simulink model "test_init"  (Simulink 10.0)
settings: Solver=FixedStepDiscrete  StartTime=0.0  StopTime=100.0  FixedStep=1  RelTol=1e-3  EnableMultiTasking=on
settings Model: Creator=kbrotman  LastModifiedBy=celit
settings DataIOCC: LimitDataPoints=on  SignalLoggingSaveFormat=ModelDataLogs  SignalLoggingName=sigsOut
settings OptimizationCC: LifeSpan=auto
settings DebuggingCC: SaveWithParameterizedLinksMsg=none  UnderspecifiedInitializationDetection=Simplified  SignalResolutionControl=TryResolveAllWithWarning  MultiTaskDSMMsg=warning  MultiTaskCondExecSysMsg=none  SFUnexpectedBacktrackingDiag=error  SFNoUnconditionalDefaultTransitionDiag=error  SFExecutionAtInitializationDiag=warning  ArithmeticOperatorsInVariantConditions=error
settings HardwareCC: ProdBitPerPointer=64  ProdBitPerSizeT=64  ProdBitPerPtrDiffT=64  ProdLargestAtomicFloat=Float  ProdIntDivRoundTo=Zero  ProdEndianess=LittleEndian  ProdWordSize=64  ProdHWDeviceType=Intel->x86-64 (Windows64)  TargetBitPerPointer=64  TargetBitPerSizeT=64  TargetBitPerPtrDiffT=64  TargetLongLongMode=on  TargetIntDivRoundTo=Zero  TargetEndianess=LittleEndian  TargetWordSize=64  TargetHWDeviceType=MATLAB Host  ProdEqTarget=off
settings SFSimCC: SimUseLocalCustomCode=on  CustomCodeUndefinedFunction=FilterOut
settings RTWCC: Description=Create Visual C/C++ Solution File for Simulink Coder  GenCodeOnly=on  TemplateMakefile=RTW.MSVCBuild  RTWUseLocalCustomCode=on  TargetLang=C++
settings CodeAppCC: StateflowObjectComments=off
settings GRTTargetCC: TargetLangStandard=C++03 (ISO)  CombineOutputUpdateFcns=on  MultiInstanceERTCode=on  CodeInterfacePackaging=C++ class  GRTInterface=off
settings CPPComponent: GenerateDestructor=on  GenerateExternalIOAccessMethods=None  ParameterMemberVisibility=private  InternalMemberVisibility=private  GenerateParameterAccessMethods=None  GenerateInternalMemberAccessMethods=None  UseOperatorNewForModelRefRegistration=off

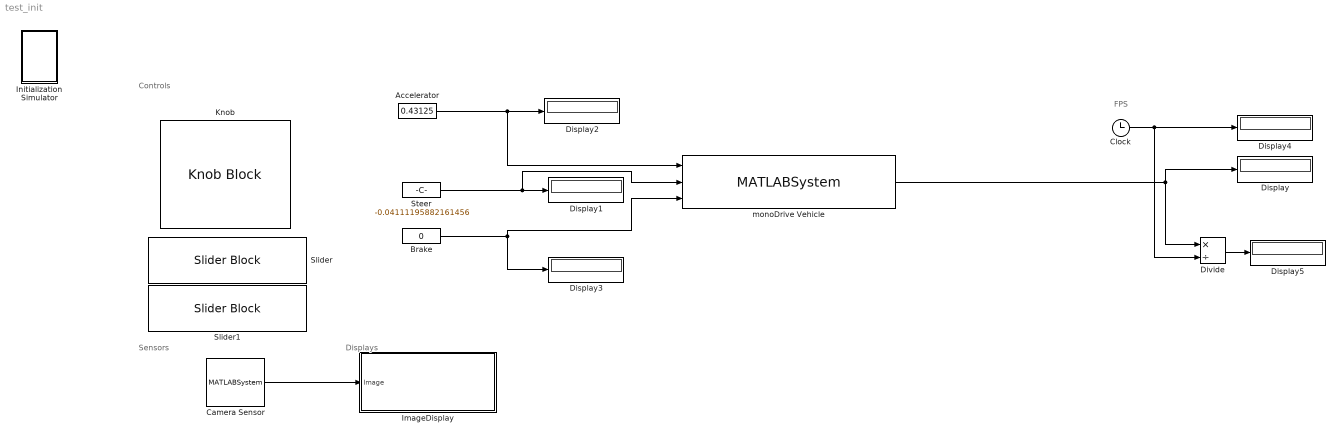
== system test_init ==
  note: Displays
  note: FPS
  note: Controls
  note: Sensors
  Accelerator : Constant  Value=0.43125  OutDataTypeStr=double  SampleTime=-1
  Brake : Constant  Value=0  OutDataTypeStr=double  SampleTime=-1
  Camera Sensor : MATLABSystem  Priority=2  System=CameraSensor  config_path=../configurations/camera.json  server_port=8999  HEADER_CONTROL=uint32( hex2dec( '6d6f6e6f' ) )  HEADER_RESPONSE=uint32( hex2dec( '6f6e6f6d' ) )  SampleTime=1  OffsetTime=0  TickTime=0.1  SimulateUsing=Interpreted execution
      mask Type: CameraSensor
      mask Display:
      | disp('CameraSensor');
      | port_label('output',1,'y');
  Clock : Clock
  Display{,1..5} (6 alike) : Display
  Divide : Product  Inputs=*/
  ImageDisplay : Subsystem
  Initialization Simulator : Subsystem  InitFcn=closed_loop_init  mask{init_in=}
      mask prompts: init_in "Enter Initialization Script:"
      mask Callback init_in:
      | init_script=get_param(gcb,'MaskValueString');
      | %eval(init_script);
      | %set_param(gcs,'PreLoadFcn',init_script)
      | set_param(gcs,'InitFcn',init_script)
  Knob : KnobBlock  LabelPosition=Bottom  ScaleMin=-1  ScaleMax=1  TickInterval=.25
  Slider : SliderBlock  LabelPosition=Bottom  ScaleMax=1  TickInterval=.2
  Slider1 : SliderBlock  LabelPosition=Bottom  ScaleMax=1  TickInterval=.2
  Steer : Constant  Value=-0.04111195882161456  SampleTime=-1
  monoDrive Vehicle : MATLABSystem  Priority=2  System=monoDriveVehicle  server_port=8999  HEADER_CONTROL=uint32( hex2dec( '6d6f6e6f' ) )  HEADER_RESPONSE=uint32( hex2dec( '6f6e6f6d' ) )  SampleTime=1  OffsetTime=0  TickTime=1  SimulateUsing=Interpreted execution
      mask Type: monoDriveVehicle
      mask Display:
      | disp('monoDriveVehicle');
      | port_label('input',1,'forward_amount');
      | port_label('input',2,'right_amount');
      | port_label('input',3,'brake_amount');
      | port_label('output',1,'Count');
  wires:
  Clock/1 -> Divide/2, Display4/1
  Divide/1 -> Display5/1
  monoDrive Vehicle/1 -> Display/1, Divide/1
  Steer/1 -> monoDrive Vehicle/2, Display1/1
  Camera Sensor/1 -> ImageDisplay/1(Image)
  Brake/1 -> Display3/1, monoDrive Vehicle/3
  Accelerator/1 -> monoDrive Vehicle/1, Display2/1

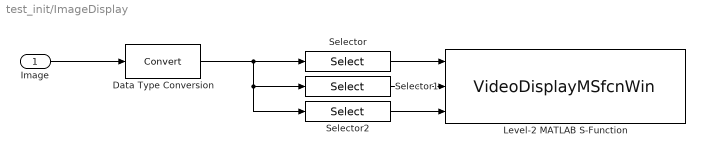
== system test_init/ImageDisplay ==
  Image : Inport
  Data Type Conversion : DataTypeConversion
  Level-2 MATLAB S-Function : M-S-Function  FunctionName=VideoDisplayMSfcnWin  Parameters=1
  Selector : Selector  NumberOfDimensions=3  InputPortWidth=3  IndexOptions=Select all,Select all,Index vector (dialog)  Indices=[1 3],1,1  OutputSizes=1,1,1
  Selector1 : Selector  NumberOfDimensions=3  InputPortWidth=3  IndexOptions=Select all,Select all,Index vector (dialog)  Indices=[1 3],1,2  OutputSizes=1,1,1
  Selector2 : Selector  NumberOfDimensions=3  InputPortWidth=3  IndexOptions=Select all,Select all,Index vector (dialog)  Indices=[1 3],1,3  OutputSizes=1,1,1
  wires:
  Data Type Conversion/1 -> Selector2/1, Selector1/1, Selector/1
  Image/1 -> Data Type Conversion/1
  Selector1/1 -> Level-2 MATLAB S-Function/2
  Selector2/1 -> Level-2 MATLAB S-Function/3
  Selector/1 -> Level-2 MATLAB S-Function/1

== system test_init/Initialization Simulator ==
